simulink model "Lab2_signal_demodulator"  (R2023b)
settings: Solver=VariableStepAuto  StartTime=0.0  StopTime=10.0  RelTol=1e-3
settings Model: Creator=Mithil Jogi  LastModifiedBy=Mithil Jogi

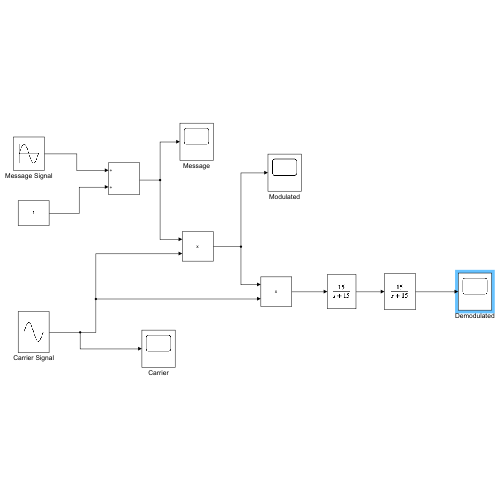
[thumbnail: Simulink's stored preview of the top-level diagram]
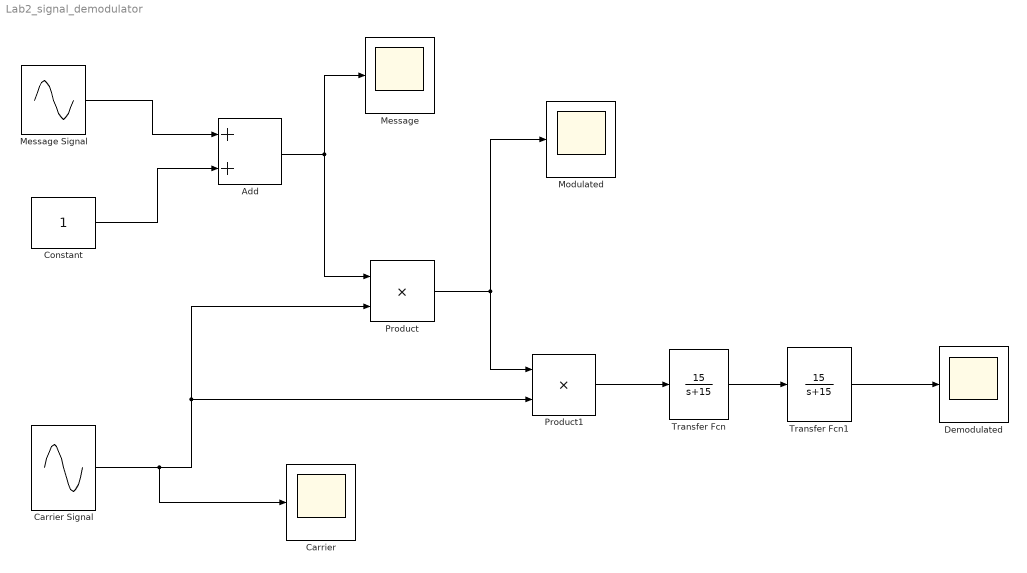
== system Lab2_signal_demodulator ==
  Add : Sum
  Carrier : Scope
  Carrier Signal : Sin  Amplitude=3  Frequency=50  SampleTime=0
  Constant : Constant
  Demodulated : Scope
  Message : Scope
  Message Signal : Sin  Amplitude=3  Frequency=5  SampleTime=0
  Modulated : Scope
  Product : Product
  Product1 : Product
  Transfer Fcn : TransferFcn  Numerator=[15]  Denominator=[1 15]
  Transfer Fcn1 : TransferFcn  Numerator=[15]  Denominator=[1 15]
  wires:
  Add/1 -> Message/1, Product/1
  Carrier Signal/1 -> Carrier/1, Product1/2, Product/2
  Product/1 -> Product1/1, Modulated/1
  Product1/1 -> Transfer Fcn/1
  Transfer Fcn/1 -> Transfer Fcn1/1
  Transfer Fcn1/1 -> Demodulated/1
  Message Signal/1 -> Add/1
  Constant/1 -> Add/2
